simulink model "feedbacklin"  (R2020b)
settings: Solver=VariableStepAuto  StartTime=0.0  StopTime=40  RelTol=1e-3
values from neighbouring files (symbols this model uses):
  Ax = 25    [main.m]
  Ay = 25    [main.m]
  d2x = sym('d2x', 'real')    [AL.m]    (also in FL.m; main.m = 0)
  d2z = sym('d2z', 'real')    [AL.m]    (also in FL.m; main.m = 0.0979)
  dgx = sym('dgx', 'real')    [AL.m]    (also in FL.m; main.m = 0)
  gravity = sym('gravity','real')    [AL.m]    (also in FL.m; main.m = 9.81)
  J1 = sym('J1', 'real')    [AL.m]    (also in FL.m; main.m = 0.0154)
  J2 = sym('J2', 'real')    [AL.m]    (also in FL.m; main.m = 0.0011)
  Jm = sym('Jm', 'real')    [AL.m]    (also in FL.m; main.m = 0.4101)
  m1 = sym('m1','real')    [AL.m]    (also in FL.m; main.m = 1.309)
  m2 = sym('m2','real')    [AL.m]    (also in FL.m; main.m = 0.098)
  mM = sym('mM','real')    [AL.m]    (also in FL.m = sym('m','real'); main.m = 0.06)
  selector = select(1)    [main.m]    (also in select.m = input('? '))
  wx = 0.16    [main.m]
  wy = 0.16    [main.m]
(part 2 of 2)

== matlab function feedbacklin/New coordinate z ==
  data: zn input; zeta output; m2 parameter; d2x parameter; d2z parameter; gravity parameter; m1 parameter; mM parameter; J2 parameter; Jm parameter
function zeta = coordinate(zn, m2, d2x, d2z, gravity, m1, mM, J2, Jm)

% State variables
pc1x = zn(1);
pc1z = zn(2);
pc1x_dot = zn(3);
pc1z_dot = zn(4);
theta1 = zn(5);
theta1_dot = zn(6);
theta12 = zn(7);
theta12_dot = zn(8);
ut = zn(9);
tau = zn(10);
w1 = zn(11);
w2 = zn(12);

% Parameters
d2 = [d2x; d2z];
mb = J2 + Jm + m2*norm(d2)^2;
ms = m1 + m2 + mM;

% New state variables (12x1)
zeta = [
 
                                                                                                                                                                                                                                                                                                                                                                                                                                                                                                                                                                                                                                                                                                                                                                                                                                                                                                                                                                                                                                                                                                                                                                                                                                                                                                                                                                                                                                                                                                             pc1x
                                                                                                                                                                                                                                                                                                                                                                                                                                                                                                                                                                                                                                                                                                                                                                                                                                                                                                                                                                                                                                                                                                                                                                                                                                                                                                                                                                                                                                                                                                         pc1x_dot
                                                                                                                                                                                                                                                                                                                                                                                                                                                                                                                                                                                                                                                                                                                                                                                                   -(d2x^2*m2^2*ut*sin(theta1) + d2z^2*m2^2*ut*sin(theta1) - d2x^2*m2^2*ut*sin(theta1 - 2*theta12) + d2z^2*m2^2*ut*sin(theta1 - 2*theta12) - 2*mb*ms*ut*sin(theta1) - d2x^2*gravity*m2^2*ms - d2z^2*gravity*m2^2*ms - d2x^2*gravity*m2^2*ms*sin(2*theta12) + d2z^2*gravity*m2^2*ms*sin(2*theta12) - 2*d2x*d2z*m2^2*ut*cos(theta1 - 2*theta12) + 2*d2x*m2*ms*tau*cos(theta12) + 2*d2z*m2*ms*tau*sin(theta12) - d2x^2*gravity*m2^2*ms*cos(2*theta12) + d2z^2*gravity*m2^2*ms*cos(2*theta12) + 2*d2x*d2z*gravity*m2^2*ms*cos(2*theta12) - 2*d2x*d2z*gravity*m2^2*ms*sin(2*theta12) + 2*d2x*m2*mb*ms*theta12_dot^2*cos(theta12) + 2*d2z*m2*mb*ms*theta12_dot^2*sin(theta12))/(2*ms*(d2x^2*m2^2 + d2z^2*m2^2 - mb*ms))
        (w1*(d2x^2*m2^2*sin(theta1 - 2*theta12) - d2z^2*m2^2*sin(theta1 - 2*theta12) + 2*mb*ms*sin(theta1) - d2x^2*m2^2*sin(theta1) - d2z^2*m2^2*sin(theta1) + 2*d2x*d2z*m2^2*cos(theta1 - 2*theta12)))/(2*ms*(d2x^2*m2^2 + d2z^2*m2^2 - mb*ms)) - (m2*w2*(d2x*cos(theta12) + d2z*sin(theta12)))/(d2x^2*m2^2 + d2z^2*m2^2 - mb*ms) + (m2*theta12_dot*(d2z^2*m2*ut*cos(theta1 - 2*theta12) - d2x^2*m2*ut*cos(theta1 - 2*theta12) - d2z*ms*tau*cos(theta12) + d2x*ms*tau*sin(theta12) + 2*d2x*d2z*m2*ut*sin(theta1 - 2*theta12) - d2z*mb*ms*theta12_dot^2*cos(theta12) + d2x*mb*ms*theta12_dot^2*sin(theta12) + d2x^2*gravity*m2*ms*cos(2*theta12) - d2z^2*gravity*m2*ms*cos(2*theta12) - d2x^2*gravity*m2*ms*sin(2*theta12) + d2z^2*gravity*m2*ms*sin(2*theta12) + 2*d2x*d2z*gravity*m2*ms*cos(2*theta12) + 2*d2x*d2z*gravity*m2*ms*sin(2*theta12)))/(ms*(d2x^2*m2^2 + d2z^2*m2^2 - mb*ms)) - (theta1_dot*ut*(d2x^2*m2^2*cos(theta1) - 2*mb*ms*cos(theta1) + d2z^2*m2^2*cos(theta1) - d2x^2*m2^2*cos(theta1 - 2*theta12) + d2z^2*m2^2*cos(theta1 - 2*theta12) + 2*d2x*d2z*m2^2*sin(theta1 - 2*theta12)))/(2*ms*(d2x^2*m2^2 + d2z^2*m2^2 - mb*ms)) - (2*m2*mb*theta12_dot*(d2x*cos(theta12) + d2z*sin(theta12))*(d2z*m2*ut*cos(theta1 - theta12) - d2x^2*m2^2*theta12_dot^2 - d2z^2*m2^2*theta12_dot^2 - ms*tau + d2x*m2*ut*sin(theta1 - theta12) + d2x*gravity*m2*ms*cos(theta12) - d2z*gravity*m2*ms*cos(theta12) + d2x*gravity*m2*ms*sin(theta12) + d2z*gravity*m2*ms*sin(theta12)))/(d2x^2*m2^2 + d2z^2*m2^2 - mb*ms)^2
                                                                                                                                                                                                                                                                                                                                                                                                                                                                                                                                                                                                                                                                                                                                                                                                                                                                                                                                                                                                                                                                                                                                                                                                                                                                                                                                                                                                                                                                                                             pc1z
                                                                                                                                                                                                                                                                                                                                                                                                                                                                                                                                                                                                                                                                                                                                                                                                                                                                                                                                                                                                                                                                                                                                                                                                                                                                                                                                                                                                                                                                                                         pc1z_dot
                                                                                                                                                                                                                                                                                                                                                                                                                                                                                                                                                                                                                                                                                                                                                                                (d2z^2*m2^2*ut*cos(theta1 - 2*theta12) - d2x^2*m2^2*ut*cos(theta1) - d2z^2*m2^2*ut*cos(theta1) - d2x^2*m2^2*ut*cos(theta1 - 2*theta12) - 2*gravity*mb*ms^2 + 2*mb*ms*ut*cos(theta1) + d2x^2*gravity*m2^2*ms + d2z^2*gravity*m2^2*ms - d2x^2*gravity*m2^2*ms*sin(2*theta12) + d2z^2*gravity*m2^2*ms*sin(2*theta12) + 2*d2x*d2z*m2^2*ut*sin(theta1 - 2*theta12) - 2*d2z*m2*ms*tau*cos(theta12) + 2*d2x*m2*ms*tau*sin(theta12) + d2x^2*gravity*m2^2*ms*cos(2*theta12) - d2z^2*gravity*m2^2*ms*cos(2*theta12) + 2*d2x*d2z*gravity*m2^2*ms*cos(2*theta12) + 2*d2x*d2z*gravity*m2^2*ms*sin(2*theta12) - 2*d2z*m2*mb*ms*theta12_dot^2*cos(theta12) + 2*d2x*m2*mb*ms*theta12_dot^2*sin(theta12))/(2*ms*(d2x^2*m2^2 + d2z^2*m2^2 - mb*ms))
        (w1*(2*mb*ms*cos(theta1) - d2x^2*m2^2*cos(theta1) - d2z^2*m2^2*cos(theta1) - d2x^2*m2^2*cos(theta1 - 2*theta12) + d2z^2*m2^2*cos(theta1 - 2*theta12) + 2*d2x*d2z*m2^2*sin(theta1 - 2*theta12)))/(2*ms*(d2x^2*m2^2 + d2z^2*m2^2 - mb*ms)) - (m2*w2*(d2z*cos(theta12) - d2x*sin(theta12)))/(d2x^2*m2^2 + d2z^2*m2^2 - mb*ms) + (m2*theta12_dot*(d2z^2*m2*ut*sin(theta1 - 2*theta12) - d2x^2*m2*ut*sin(theta1 - 2*theta12) + d2x*ms*tau*cos(theta12) + d2z*ms*tau*sin(theta12) - 2*d2x*d2z*m2*ut*cos(theta1 - 2*theta12) + d2x*mb*ms*theta12_dot^2*cos(theta12) + d2z*mb*ms*theta12_dot^2*sin(theta12) - d2x^2*gravity*m2*ms*cos(2*theta12) + d2z^2*gravity*m2*ms*cos(2*theta12) - d2x^2*gravity*m2*ms*sin(2*theta12) + d2z^2*gravity*m2*ms*sin(2*theta12) + 2*d2x*d2z*gravity*m2*ms*cos(2*theta12) - 2*d2x*d2z*gravity*m2*ms*sin(2*theta12)))/(ms*(d2x^2*m2^2 + d2z^2*m2^2 - mb*ms)) + (theta1_dot*ut*(d2x^2*m2^2*sin(theta1 - 2*theta12) - d2z^2*m2^2*sin(theta1 - 2*theta12) - 2*mb*ms*sin(theta1) + d2x^2*m2^2*sin(theta1) + d2z^2*m2^2*sin(theta1) + 2*d2x*d2z*m2^2*cos(theta1 - 2*theta12)))/(2*ms*(d2x^2*m2^2 + d2z^2*m2^2 - mb*ms)) - (2*m2*mb*theta12_dot*(d2z*cos(theta12) - d2x*sin(theta12))*(d2z*m2*ut*cos(theta1 - theta12) - d2x^2*m2^2*theta12_dot^2 - d2z^2*m2^2*theta12_dot^2 - ms*tau + d2x*m2*ut*sin(theta1 - theta12) + d2x*gravity*m2*ms*cos(theta12) - d2z*gravity*m2*ms*cos(theta12) + d2x*gravity*m2*ms*sin(theta12) + d2z*gravity*m2*ms*sin(theta12)))/(d2x^2*m2^2 + d2z^2*m2^2 - mb*ms)^2
                                                                                                                                                                                                                                                                                                                                                                                                                                                                                                                                                                                                                                                                                                                                                                                                                                                                                                                                                                                                                                                                                                                                                                                                                                                                                                                                                                                                                                                                                                          theta12
                                                                                                                                                                                                                                                                                                                                                                                                                                                                                                                                                                                                                                                                                                                                                                                                                                                                                                                                                                                                                                                                                                                                                                                                                                                                                                                                                                                                                                                                                                      theta12_dot
                                                                                                                                                                                                                                                                                                                                                                                                                                                                                                                                                                                                                                                                                                                                                                                                                                                                                                                                                                                                                                                                                                                                                                                                         (d2z*m2*ut*cos(theta1 - theta12) - d2x^2*m2^2*theta12_dot^2 - d2z^2*m2^2*theta12_dot^2 - ms*tau + d2x*m2*ut*sin(theta1 - theta12) + d2x*gravity*m2*ms*cos(theta12) - d2z*gravity*m2*ms*cos(theta12) + d2x*gravity*m2*ms*sin(theta12) + d2z*gravity*m2*ms*sin(theta12))/(d2x^2*m2^2 + d2z^2*m2^2 - mb*ms)
                                                                                                                                                                                                                                                                                                                                                                                                                                                                                                                                                                                                                                                        (m2*w1*(d2z*cos(theta1 - theta12) + d2x*sin(theta1 - theta12)))/(d2x^2*m2^2 + d2z^2*m2^2 - mb*ms) - (ms*w2)/(d2x^2*m2^2 + d2z^2*m2^2 - mb*ms) + (m2*theta12_dot*(d2z*ut*sin(theta1 - theta12) - d2x*ut*cos(theta1 - theta12) + d2x*gravity*ms*cos(theta12) + d2z*gravity*ms*cos(theta12) - d2x*gravity*ms*sin(theta12) + d2z*gravity*ms*sin(theta12)))/(d2x^2*m2^2 + d2z^2*m2^2 - mb*ms) - (2*m2^2*theta12_dot*(d2x^2 + d2z^2)*(d2z*m2*ut*cos(theta1 - theta12) - d2x^2*m2^2*theta12_dot^2 - d2z^2*m2^2*theta12_dot^2 - ms*tau + d2x*m2*ut*sin(theta1 - theta12) + d2x*gravity*m2*ms*cos(theta12) - d2z*gravity*m2*ms*cos(theta12) + d2x*gravity*m2*ms*sin(theta12) + d2z*gravity*m2*ms*sin(theta12)))/(d2x^2*m2^2 + d2z^2*m2^2 - mb*ms)^2 + (m2*theta1_dot*ut*(d2x*cos(theta1 - theta12) - d2z*sin(theta1 - theta12)))/(d2x^2*m2^2 + d2z^2*m2^2 - mb*ms)];

== matlab function feedbacklin/Controller ==
  data: ref input; zi input; v_aux output; lambda parameter
function v_aux  = poles_placement(ref, zi, lambda)


% Reference trajectories
pc1_x = ref(1);
pc1_xd1 = ref(2);
pc1_xd2 = ref(3);
pc1_xd3 = ref(4);
pc1_xd4 = ref(5); 
pc1_z = ref(6);
pc1_zd1 = ref(7);
pc1_zd2 = ref(8);
pc1_zd3 = ref(9);
pc1_zd4 = ref(10);
theta = ref(11);
theta_d1 = ref(12);
theta_d2 = ref(13);
theta_d3 = ref(14);
theta_d4 = ref(15);

% Control coefficients
lambda1 = lambda(1);
lambda2 = lambda(2);
lambda3 = lambda(3);
lambda4 = lambda(4);
lambda5 = lambda(5);
lambda6 = lambda(6);
lambda7 = lambda(7);
lambda8 = lambda(8);
lambda9 = lambda(9);
lambda10 = lambda(10);
lambda11 = lambda(11);
lambda12 = lambda(12);

% Control law
v_aux = zeros(3,1);
    v_aux(1) = pc1_xd4 - lambda3*(zi(3)-pc1_xd2) - lambda2*(zi(2)-pc1_xd1) - lambda1*(zi(1)-pc1_x) - lambda4*(zi(4)-pc1_xd3);
    v_aux(2) = pc1_zd4 - lambda7*(zi(7)-pc1_zd2) - lambda6*(zi(6)-pc1_zd1) - lambda5*(zi(5)-pc1_z) - lambda8*(zi(8)-pc1_zd3);
    v_aux(3) = theta_d4 - lambda11*(zi(11)-theta_d2) - lambda10*(zi(10)-theta_d1) - lambda9*(zi(9)-theta) - lambda12*(zi(12)-theta_d3);


% Errorors in Trajectory Tracking:
ex = zi(1) - pc1_x;
ey = zi(5) - pc1_z;
et = zi(12) - theta;

end
